simulink model "Sfunctiontest_20220810"  (R2021a)
settings: Solver=VariableStepAuto  StartTime=0.0  StopTime=360  RelTol=1e-3
undefined symbols (not defined in the file or in its folder): newDymolaGui
libraries: simulink x1
settings Model: Creator=jason  LastModifiedBy=jason

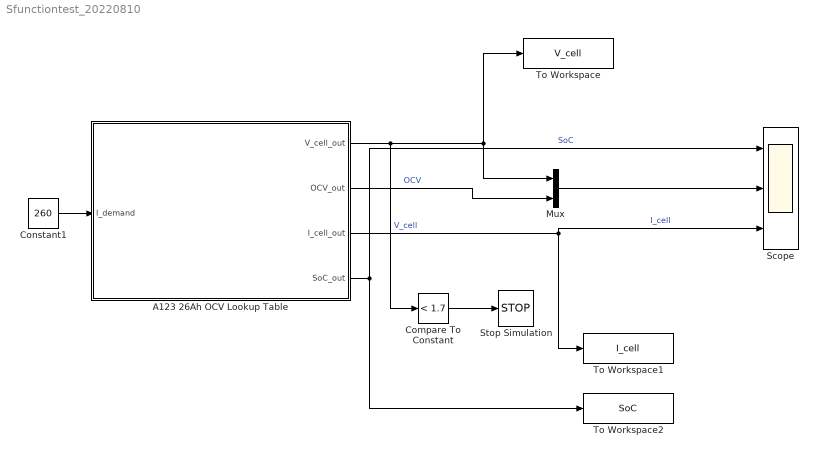
== system Sfunctiontest_20220810 ==
  A123 26Ah OCV Lookup Table : Subsystem  Tag=11-Aug-2022 00:13:00#9058
      mask help:
      | Dymola block.
      | A dymola block allows acausal physical modeling.
      | See Dymola manual for usage.
      settings: CopyFcn=newDymolaGui('11-Aug-2022 00:13:00#9058','Copy');  DeleteFcn=if exist('newDymolaGui') newDymolaGui('Sfunctiontest_20220810/A123 26Ah OCV Lookup Table','Delete'); end;  NameChangeFcn=newDymolaGui('11-Aug-2022 00:13:00#9058','Copy');  OpenFcn=newDymolaGui('Sfunctiontest_20220810/A123 26Ah OCV Lookup Table','Init');
      mask Display: image(imread('Dymola.bmp'),[.2,.2,.6,.6])
  Compare To Constant : simulink/Logic and Bit Operations/Compare To Constant  relop=<  const=1.7  OutDataTypeStr=boolean
  Constant1 : Constant  Value=260
  Mux : Mux  Inputs=2
  Scope : Scope  NumInputPorts=3
  Stop Simulation : Stop
  To Workspace : ToWorkspace  VariableName=V_cell  SampleTime=-1
  To Workspace1 : ToWorkspace  VariableName=I_cell  SampleTime=-1
  To Workspace2 : ToWorkspace  VariableName=SoC  SampleTime=-1
  wires:
  A123 26Ah OCV Lookup Table/1(V_cell_out) -> Compare To Constant/1, To Workspace/1, Mux/1  "V_cell"
  A123 26Ah OCV Lookup Table/3(I_cell_out) -> To Workspace1/1, Scope/3  "I_cell"
  Constant1/1 -> A123 26Ah OCV Lookup Table/1(I_demand)
  Compare To Constant/1 -> Stop Simulation/1
  A123 26Ah OCV Lookup Table/2(OCV_out) -> Mux/2  "OCV"
  Mux/1 -> Scope/2
  A123 26Ah OCV Lookup Table/4(SoC_out) -> Scope/1, To Workspace2/1  "SoC"

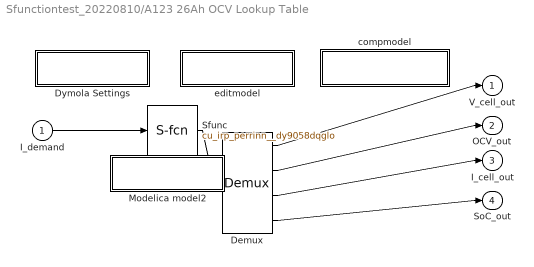
== system Sfunctiontest_20220810/A123 26Ah OCV Lookup Table ==
  I_demand : Inport
  Demux : Demux  Outputs=[1;1;1;1]
  Dymola Settings : Subsystem  mask{ModelName=CU_IRP_perrinn_battery.Electrical.Batteries.Electro_therml_3D.ECM_2RC_A123_26Ah, MoFileName=C:/Users/jason/OneDrive - The Hong Kong Polytechnic University/Cranfield Studies/4 Course Projects/IRP Battery/dymola_git/CU_IRP_perrinn_battery/Electrical/Batteries/Electro_therml_3D, dSpace=, BusConnector=0, ResultFile=[], ResultFileOnline=[], ResultDt=[], Libs=:, bigobj=[], ImportFolder=[], guimode=[], ModelName2=[], forRuntime=[], MEXLoad=[], omitDescription=[], ResultName=cu_irp_perrinn__dy9058dqglo}
      mask prompts: ModelName "Name of Dymola model"; MoFileName "File Name (including .mo)"; ResultFile "Create Result"; ResultFileOnline "Load result"; ResultDt "Result min dt"; Libs "Used Libraries"; bigobj "Compiler flag /bigobj"; ImportFolder "Import folder"; guimode "GUI mode flag"; ModelName2 "Model name for import mode"; forRuntime "Runtime export"; MEXLoad "Compiled S-function"; omitDescription "Omit description strings"; ResultName "Name of result file"
      mask Display: disp('Dymola Settings');
  Modelica model2 : Subsystem
      mask Display: disp('Change parameters');
  Sfunc : S-Function  Tag=9058dqglo  FunctionName=cu_irp_perrinn__dy9058dqglo  Parameters=[R0_R;R1_R;C2_C;C2_IC;C2_UIC;R2_R;C1_C;C1_IC;C1_UIC;DoD_OCV_verboseRead;columb_Counting_integrato11;columb_Counting_integrato12;columb_Counting_add_k1;columb_Counting_add_k2;columb_Counting_const_k;columb_Counting_gain_k;Ah_design_k],[C2_vinternal;C1_vinternal;columb_Counting_integrato20]  PortCounts=[1;1]  SFunctionDeploymentMode=off  EnableBusSupport=off  mask{R0_R=0.0015, R1_R=0.0047, C2_C=2932, C2_IC=0, C2_UIC=0, R2_R=0.0003, C1_C=180000, C1_IC=0, C1_UIC=0, DoD_OCV_verboseRead=1, columb_Counting_integrato11=1, columb_Counting_integrato12=0, columb_Counting_add_k1=-1, columb_Counting_add_k2=1, columb_Counting_const_k=1, columb_Counting_gain_k=3600, Ah_design_k=16.8, C2_vinternal=0, C1_vinternal=0, columb_Counting_integrato20=0}
      mask prompts: R0_R "R0.R"; R1_R "R1.R"; C2_C "C2.C"; C2_IC "C2.IC"; C2_UIC "C2.UIC"; R2_R "R2.R"; C1_C "C1.C"; C1_IC "C1.IC"; C1_UIC "C1.UIC"; DoD_OCV_verboseRead "DoD_OCV.verboseRead"; columb_Counting_integrato11 "columb_Counting.integrator.k"; columb_Counting_integrato12 "columb_Counting.integrator.y_start"; columb_Counting_add_k1 "columb_Counting.add.k1"; columb_Counting_add_k2 "columb_Counting.add.k2"; columb_Counting_const_k "columb_Counting.const.k"; columb_Counting_gain_k "columb_Counting.gain.k"; Ah_design_k "Ah_design.k"; C2_vinternal "C2.vinternal"; C1_vinternal "C1.vinternal"; columb_Counting_integrato20 "columb_Counting.integrator.y"
      mask Display: image(imread('Dymola.bmp'))
  compmodel : Subsystem  InitFcn=newDymolaGui('Sfunctiontest_20220810/A123 26Ah OCV Lookup Table','Verify');
      settings: OpenFcn=compileModelica('Sfunctiontest_20220810/A123 26Ah OCV Lookup Table');
      mask Display: disp('Compile Modelica model');
  editmodel : Subsystem
      settings: OpenFcn=editModelica('Sfunctiontest_20220810/A123 26Ah OCV Lookup Table');
      mask Display: disp('Edit Modelica model');
  V_cell_out : Outport
  OCV_out : Outport  Port=2
  I_cell_out : Outport  Port=3
  SoC_out : Outport  Port=4
  wires:
  Sfunc/1 -> Demux/1
  Demux/1 -> V_cell_out/1
  Demux/2 -> OCV_out/1
  Demux/3 -> I_cell_out/1
  Demux/4 -> SoC_out/1
  I_demand/1 -> Sfunc/1

== system Sfunctiontest_20220810/A123 26Ah OCV Lookup Table/Dymola Settings ==

== system Sfunctiontest_20220810/A123 26Ah OCV Lookup Table/Modelica model2 ==

== system Sfunctiontest_20220810/A123 26Ah OCV Lookup Table/compmodel ==

== system Sfunctiontest_20220810/A123 26Ah OCV Lookup Table/editmodel ==
